simulink library "ad_mem_scalar"  (R2017a)
settings: Solver=VariableStepAuto  StartTime=0.0  StopTime=10.0  RelTol=1e-3
libraries: autodiff x9, ad_mem_base x2, ad_mem_scalar x2
settings Model: Creator=eruffaldi  LastModifiedBy=eruffaldi

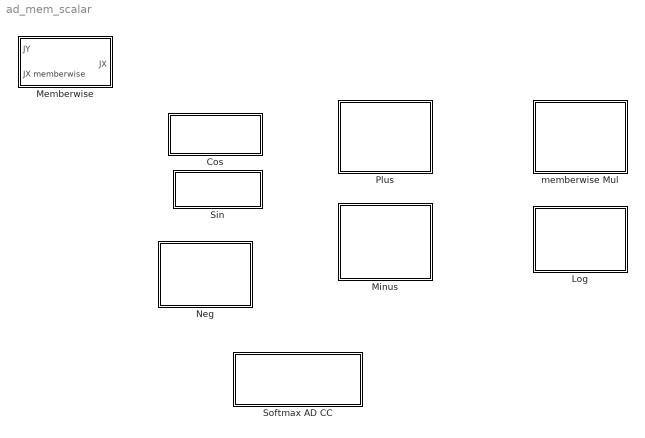
== system ad_mem_scalar ==
  Cos : Subsystem
      mask Display: disp('cos(x)');
  Log : Subsystem
  Memberwise : Subsystem
  "Minus " : Subsystem
  Neg : Subsystem
  Plus : Subsystem
  Sin : Subsystem
      mask Display: disp('sin(x)');
  Softmax AD CC : Subsystem
      mask Display: image('softmax.png');
  memberwise Mul : Subsystem

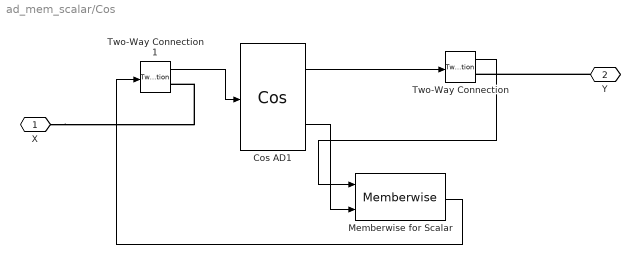
== system ad_mem_scalar/Cos ==
  Cos AD1 : ad_mem_base/Cos  SystemSampleTime=-1
      settings: SourceProductName=AutoDiff
  Memberwise for Scalar : ad_mem_scalar/Memberwise
  Two-Way Connection : TwoWayConnection
  Two-Way Connection1 : TwoWayConnection
  X : PMIOPort  Port=1  Side=Left
  Y : PMIOPort  Port=2  Side=Right
  wires:
  Two-Way Connection1/1 -> Cos AD1/1
  Cos AD1/1 -> Two-Way Connection/1
  Cos AD1/2 -> Memberwise for Scalar/2
  Two-Way Connection/1 -> Memberwise for Scalar/1
  Memberwise for Scalar/1 -> Two-Way Connection1/1
  connections:
  Y/RConn1 -- Two-Way Connection/RConn1
  X/RConn1 -- Two-Way Connection1/RConn1

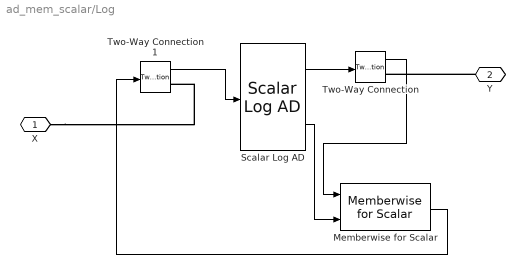
== system ad_mem_scalar/Log ==
  Memberwise for Scalar : autodiff/Common/Memberwise for Scalar
      settings: SourceProductName=AutoDiff
  Scalar Log AD : autodiff/Memberwise Base/Scalar Log AD
      settings: SourceProductName=AutoDiff
  Two-Way Connection : TwoWayConnection
  Two-Way Connection1 : TwoWayConnection
  X : PMIOPort  Port=1  Side=Left
  Y : PMIOPort  Port=2  Side=Right
  wires:
  Scalar Log AD/1 -> Two-Way Connection/1
  Two-Way Connection1/1 -> Scalar Log AD/1
  Two-Way Connection/1 -> Memberwise for Scalar/1
  Scalar Log AD/2 -> Memberwise for Scalar/2
  Memberwise for Scalar/1 -> Two-Way Connection1/1
  connections:
  Y/RConn1 -- Two-Way Connection/RConn1
  X/RConn1 -- Two-Way Connection1/RConn1

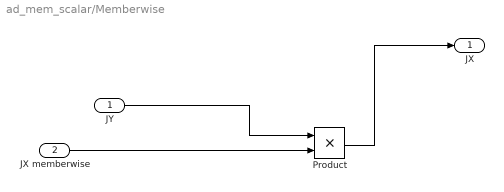
== system ad_mem_scalar/Memberwise ==
  JY : Inport
  JX memberwise : Inport  Port=2
  Product : Product
  JX : Outport
  wires:
  Product/1 -> JX/1
  JX memberwise/1 -> Product/2
  JY/1 -> Product/1

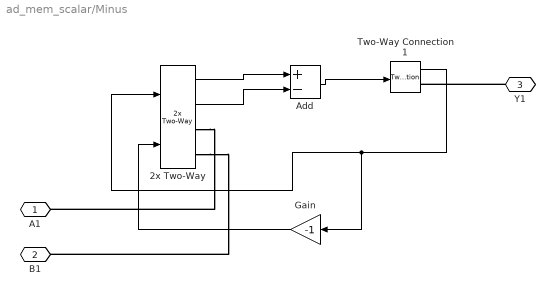
== system ad_mem_scalar/Minus  ==
  "2x Two-Way " : autodiff/Common/2x Two-Way 
      settings: SourceProductName=AutoDiff
  Add : Sum  Inputs=+-
  Gain : Gain  Gain=-1
  Two-Way Connection1 : TwoWayConnection
  A1 : PMIOPort  Port=1  Side=Left
  B1 : PMIOPort  Port=2  Side=Left
  Y1 : PMIOPort  Port=3  Side=Right
  wires:
  "2x Two-Way "/1 -> Add/1
  Two-Way Connection1/1 -> "2x Two-Way "/1, Gain/1
  Add/1 -> Two-Way Connection1/1
  Gain/1 -> "2x Two-Way "/2
  "2x Two-Way "/2 -> Add/2
  connections:
  Y1/RConn1 -- Two-Way Connection1/RConn1
  "2x Two-Way "/RConn2 -- B1/RConn1
  "2x Two-Way "/RConn1 -- A1/RConn1

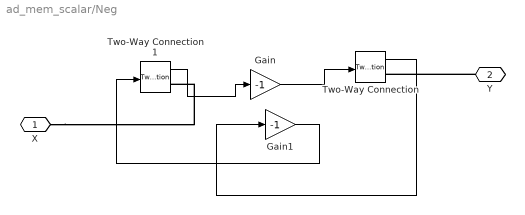
== system ad_mem_scalar/Neg ==
  Gain : Gain  Gain=-1
  Gain1 : Gain  Gain=-1
  Two-Way Connection : TwoWayConnection
  Two-Way Connection1 : TwoWayConnection
  X : PMIOPort  Port=1  Side=Left
  Y : PMIOPort  Port=2  Side=Right
  wires:
  Gain/1 -> Two-Way Connection/1
  Gain1/1 -> Two-Way Connection1/1
  Two-Way Connection1/1 -> Gain/1
  Two-Way Connection/1 -> Gain1/1
  connections:
  Y/RConn1 -- Two-Way Connection/RConn1
  X/RConn1 -- Two-Way Connection1/RConn1

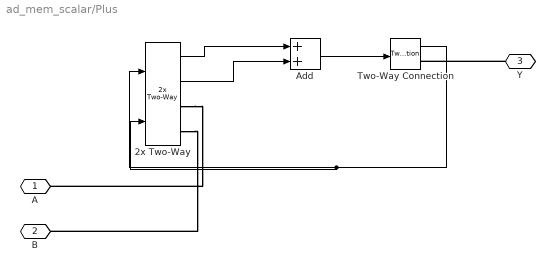
== system ad_mem_scalar/Plus ==
  "2x Two-Way " : autodiff/Common/2x Two-Way 
      settings: SourceProductName=AutoDiff
  Add : Sum
  Two-Way Connection : TwoWayConnection
  A : PMIOPort  Port=1  Side=Left
  B : PMIOPort  Port=2  Side=Left
  Y : PMIOPort  Port=3  Side=Right
  wires:
  Add/1 -> Two-Way Connection/1
  Two-Way Connection/1 -> "2x Two-Way "/1, "2x Two-Way "/2
  "2x Two-Way "/1 -> Add/1
  "2x Two-Way "/2 -> Add/2
  connections:
  Y/RConn1 -- Two-Way Connection/RConn1
  "2x Two-Way "/RConn1 -- A/RConn1
  "2x Two-Way "/RConn2 -- B/RConn1

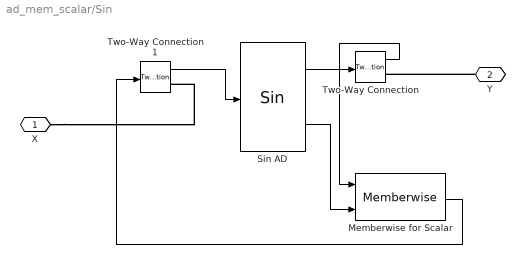
== system ad_mem_scalar/Sin ==
  Memberwise for Scalar : ad_mem_scalar/Memberwise
  Sin AD : ad_mem_base/Sin
      settings: SourceProductName=AutoDiff
  Two-Way Connection : TwoWayConnection
  Two-Way Connection1 : TwoWayConnection
  X : PMIOPort  Port=1  Side=Left
  Y : PMIOPort  Port=2  Side=Right
  wires:
  Sin AD/1 -> Two-Way Connection/1
  Two-Way Connection1/1 -> Sin AD/1
  Sin AD/2 -> Memberwise for Scalar/2
  Memberwise for Scalar/1 -> Two-Way Connection1/1
  Two-Way Connection/1 -> Memberwise for Scalar/1
  connections:
  X/RConn1 -- Two-Way Connection1/RConn1
  Y/RConn1 -- Two-Way Connection/RConn1

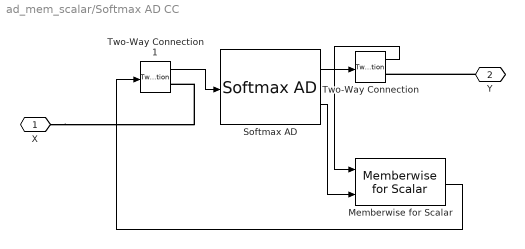
== system ad_mem_scalar/Softmax AD CC ==
  Memberwise for Scalar : autodiff/Common/Memberwise for Scalar
      settings: SourceProductName=AutoDiff
  Softmax AD : autodiff/Memberwise Base/Softmax AD  SystemSampleTime=-1
      settings: SourceProductName=AutoDiff
  Two-Way Connection : TwoWayConnection
  Two-Way Connection1 : TwoWayConnection
  X : PMIOPort  Port=1  Side=Left
  Y : PMIOPort  Port=2  Side=Right
  wires:
  Softmax AD/1 -> Two-Way Connection/1
  Two-Way Connection1/1 -> Softmax AD/1
  Two-Way Connection/1 -> Memberwise for Scalar/1
  Memberwise for Scalar/1 -> Two-Way Connection1/1
  Softmax AD/2 -> Memberwise for Scalar/2
  connections:
  Y/RConn1 -- Two-Way Connection/RConn1
  X/RConn1 -- Two-Way Connection1/RConn1

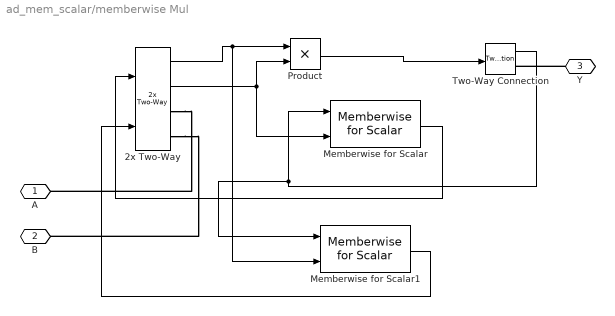
== system ad_mem_scalar/memberwise Mul ==
  "2x Two-Way " : autodiff/Common/2x Two-Way 
      settings: SourceProductName=AutoDiff
  Memberwise for Scalar : autodiff/Common/Memberwise for Scalar
      settings: SourceProductName=AutoDiff
  Memberwise for Scalar1 : autodiff/Common/Memberwise for Scalar
      settings: SourceProductName=AutoDiff
  Product : Product
  Two-Way Connection : TwoWayConnection
  A : PMIOPort  Port=1  Side=Left
  B : PMIOPort  Port=2  Side=Left
  Y : PMIOPort  Port=3  Side=Right
  wires:
  Product/1 -> Two-Way Connection/1
  Memberwise for Scalar1/1 -> "2x Two-Way "/2
  "2x Two-Way "/2 -> Product/2, Memberwise for Scalar/2
  Two-Way Connection/1 -> Memberwise for Scalar1/1, Memberwise for Scalar/1
  Memberwise for Scalar/1 -> "2x Two-Way "/1
  "2x Two-Way "/1 -> Memberwise for Scalar1/2, Product/1
  connections:
  Y/RConn1 -- Two-Way Connection/RConn1
  "2x Two-Way "/RConn1 -- A/RConn1
  "2x Two-Way "/RConn2 -- B/RConn1
